simulink model "Regulacia_JCBM_Uloha1_S"  (R2022b)
settings: Solver=VariableStepAuto  StartTime=0.0  StopTime=2  RelTol=1e-6
values from neighbouring files (symbols this model uses):
  cfi = (Ua-Ra*IN)/wN    (= 2.66063720525)    [Regulacia_JCBM_M.m]
  Jc = Jm*8    (= 2.32)    [Regulacia_JCBM_M.m]
  La = 0.0081    [Regulacia_JCBM_M.m]
  Mz = MN    (= 132)    [Regulacia_JCBM_M.m]
  Ra = 0.522    [Regulacia_JCBM_M.m]
  Ua = 420    [Regulacia_JCBM_M.m]
settings Model: Creator=hwswi  LastModifiedBy=hwswi
settings DataIOCC: ReturnWorkspaceOutputs=off

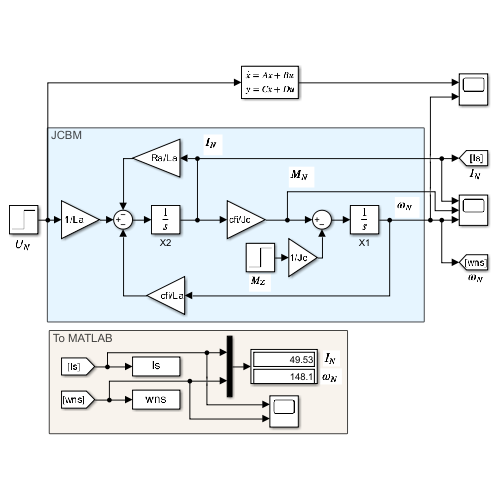
[thumbnail: Simulink's stored preview of the top-level diagram]
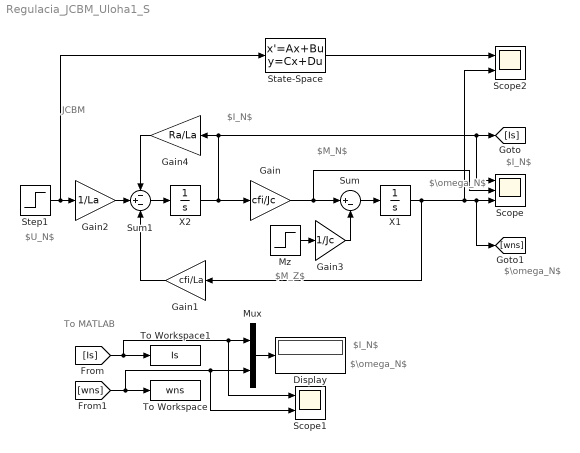
== system Regulacia_JCBM_Uloha1_S ==
  note: To MATLAB
  note: JCBM
  note: $\omega_N$
  note: $I_N$
  note: $M_N$
  note: $U_N$
  note: $I_N$
  note: $M_Z$
  note: $I_N$
  note: $\omega_N$
  note: $\omega_N$
  Display : Display
  Gain : Gain  Gain=cfi/Jc
  Gain1 : Gain  Gain=cfi/La
  Gain2 : Gain  Gain=1/La
  Gain3 : Gain  Gain=1/Jc
  Gain4 : Gain  Gain=Ra/La
  Mux : Mux  Inputs=2
  Mz : Step  After=Mz  SampleTime=0
  Scope : Scope  NumInputPorts=3
  Scope1 : Scope  NumInputPorts=2
  Scope2 : Scope  NumInputPorts=2
  State-Space : StateSpace  A=[0 (cfi/Jc);-(cfi/La) -(Ra/La)]  B=[0;1/La]  C=[1 0]  D=0  InitialCondition=0
  Step1 : Step  Time=0  After=Ua  SampleTime=0
  Sum : Sum  Inputs=|+-
  Sum1 : Sum  Inputs=-+-
  To Workspace : ToWorkspace  VariableName=wns  SaveFormat=Timeseries  SampleTime=-1
  To Workspace1 : ToWorkspace  VariableName=Is  SaveFormat=Timeseries  SampleTime=-1
  X1 : Integrator
  X2 : Integrator
  wires:
  Mux/1 -> Display/1
  Sum/1 -> X1/1
  [Is] -> To Workspace1/1, Scope1/1, Mux/1
  Gain1/1 -> Sum1/3
  Gain/1 -> Sum/1, Scope/2
  [wns] -> To Workspace/1, Scope1/2, Mux/2
  Step1/1 -> State-Space/1, Gain2/1
  X2/1 -> Gain4/1, Scope/1, [Is], Gain/1
  Sum1/1 -> X2/1
  Gain2/1 -> Sum1/2
  Gain3/1 -> Sum/2
  Gain4/1 -> Sum1/1
  X1/1 -> Scope2/2, Scope/3, [wns], Gain1/1
  Mz/1 -> Gain3/1
  State-Space/1 -> Scope2/1
